simulink model "CaseD_2"  (R2015a)
settings: Solver=ode3  SolverMode=SingleTasking  StartTime=0.0  StopTime=time  FixedStep=dt  RelTol=1e-3
values from neighbouring files (symbols this model uses):
  C = [6; 0]    [main.m]
  dt = 0.01    [main.m]
  initial_eta = [1 0 0]'    [main.m]
  initial_eta_2 = [6 5 0]'    [main.m]
  initial_eta_4 = [7 0 0]'    [main.m]
  K_p = diag([0.2,0.2,0.1])    [main.m]
  mu = 0.1    [main.m]
  P_d = [2  0 ... (first row only)    [main.m]
  R = diag(r)    [main.m]
  r = [5; 3]    [main.m]
  U_max = 1    [main.m]
  U_ref = [(0:dt:time)' [zeros(floor(1*points/6),1) ... (first row only)    [main.m]
(part 1 of 2)
settings Model: CovMetricSettings=dwe  CovHtmlReporting=off  covSaveCumulativeToWorkspaceVar=off  CovSaveSingleToWorkspaceVar=off  CovExternalEMLEnable=on  Creator=helene  LastModifiedBy=Lars
settings DataIOCC: LimitDataPoints=off  SaveFormat=Dataset
settings DebuggingCC: SFUnexpectedBacktrackingDiag=error  SFNoUnconditionalDefaultTransitionDiag=error
settings HardwareCC: ProdBitPerPointer=64  ProdLargestAtomicFloat=Float  ProdIntDivRoundTo=Zero  ProdEndianess=LittleEndian  ProdHWDeviceType=Specified
settings ModelReferenceCC: PropagateSignalLabelsOutOfModel=on
settings GRTTargetCC: TargetLangStandard=C99 (ISO)  GeneratePreprocessorConditionals=Use local settings

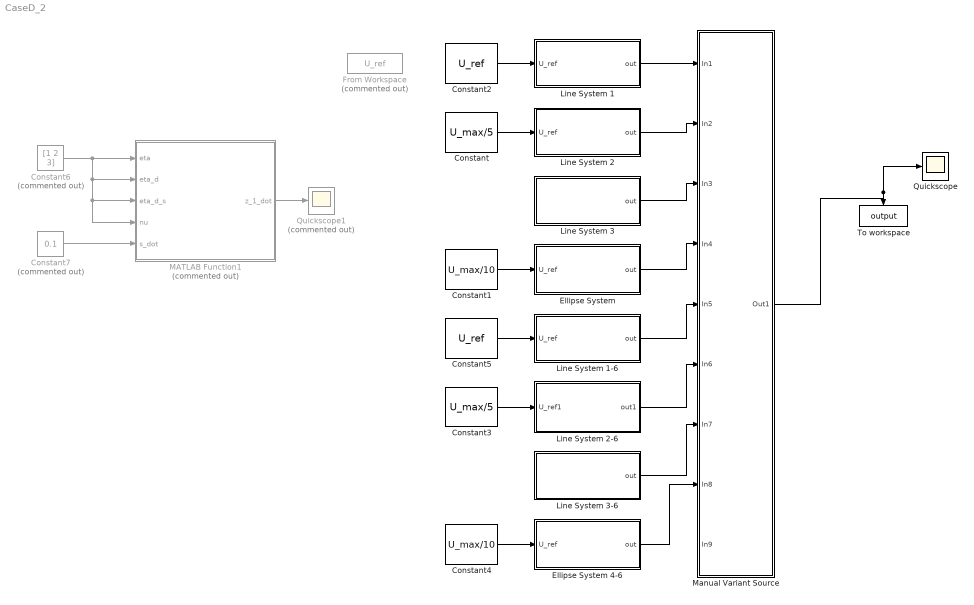
== system CaseD_2 ==
  Constant : Constant  Value=U_max/5
  Constant1 : Constant  Value=U_max/10
  Constant2 : Constant  Value=U_ref
  Constant3 : Constant  Value=U_max/5
  Constant4 : Constant  Value=U_max/10
  Constant5 : Constant  Value=U_ref
  Constant6 : Constant  Commented=on  Value=[1 2 3]
  Constant7 : Constant  Commented=on  Value=0.1
  Ellipse System : Subsystem
  Ellipse System 4-6 : Subsystem
  From Workspace : FromWorkspace  Commented=on  VariableName=U_ref  SampleTime=dt
  Line System 1 : Subsystem
  Line System 1-6 : Subsystem
  Line System 2 : Subsystem
  Line System 2-6 : Subsystem
  Line System 3 : Subsystem
  Line System 3-6 : Subsystem
  MATLAB Function1 : MATLAB Function  Commented=on  TreatAsAtomicUnit=on
      settings: PermitHierarchicalResolution=ParametersOnly
  Manual Variant Source : Subsystem  Description=Replaced Block  mask(Replaced Block){}
      mask help: This block has been replaced with an empty subsystem because it used functionality that is unavailable in Simulink R2015a.
      mask Display: fprintf('Replaced: %s\n','VariantSource')
  Quickscope : Scope
      settings: TimeRange=auto  ShowLegends=on  MaxDataPoints=5000  SaveToWorkspace=off  YMin=-2.04605  YMax=18.41446  SampleTime=-1
  Quickscope1 : Scope  Commented=on
      settings: TimeRange=auto  MaxDataPoints=5000  SaveToWorkspace=off  YMin=0.86712  YMax=2.90365  SampleTime=-1
  To workspace : ToWorkspace  VariableName=output  SampleTime=-1
      settings: StopFcn=plotting
  wires:
  Ellipse System/1(out) -> Manual Variant Source/4(In4)
  Manual Variant Source/1(Out1) -> Quickscope/1, To workspace/1
  Line System 1/1(out) -> Manual Variant Source/1(In1)
  Line System 2/1(out) -> Manual Variant Source/2(In2)
  Constant/1 -> Line System 2/1(U_ref)
  Line System 3/1(out) -> Manual Variant Source/3(In3)
  Constant1/1 -> Ellipse System/1(U_ref)
  Constant2/1 -> Line System 1/1(U_ref)
  Ellipse System 4-6/1(out) -> Manual Variant Source/8(In8)
  Line System 1-6/1(out) -> Manual Variant Source/5(In5)
  Line System 2-6/1(out1) -> Manual Variant Source/6(In6)
  Constant3/1 -> Line System 2-6/1(U_ref1)
  Line System 3-6/1(out) -> Manual Variant Source/7(In7)
  Constant4/1 -> Ellipse System 4-6/1(U_ref)
  Constant5/1 -> Line System 1-6/1(U_ref)
  Constant6/1 -> MATLAB Function1/4(nu), MATLAB Function1/3(eta_d_s), MATLAB Function1/2(eta_d), MATLAB Function1/1(eta)
  Constant7/1 -> MATLAB Function1/5(s_dot)
  MATLAB Function1/1(z_1_dot) -> Quickscope1/1

== system CaseD_2/Ellipse System ==
  U_ref : Inport
  Control law : Subsystem
  "Ellipse Mapper " : Subsystem
  Ellipse Speed Gauge : Subsystem
  Kinematic model : Subsystem
  Mux : Mux  Inputs=3
  Update Law : Subsystem
  out : Outport
  wires:
  U_ref/1 -> Ellipse Speed Gauge/1(U_ref)
  Update Law/1(s) -> Mux/3, Ellipse Speed Gauge/2(s), "Ellipse Mapper "/1(s)
  "Ellipse Mapper "/1(eta_d) -> Update Law/2(eta_d), Mux/2, Control law/4(eta_d)
  Kinematic model/1("eta ") -> Control law/1(eta), Update Law/4(eta), Mux/1
  Control law/1(nu) -> Kinematic model/1(nu)
  "Ellipse Mapper "/2(eta_d_s) -> Control law/3(eta_d_s), Update Law/3(eta_d_s)
  Ellipse Speed Gauge/1(U_s) -> Control law/2(U_s), Update Law/1(U_s)
  Mux/1 -> out/1

== system CaseD_2/Ellipse System 4-6 ==
  U_ref : Inport
  Control law1 : Subsystem
  "Ellipse Mapper " : Subsystem
  Ellipse Speed Gauge : Subsystem
  Kinematic model : Subsystem
  Mux : Mux  Inputs=3
  Update Law : Subsystem
  out : Outport
  wires:
  U_ref/1 -> Ellipse Speed Gauge/1(U_ref)
  Update Law/1(s) -> Ellipse Speed Gauge/2(s), "Ellipse Mapper "/1(s), Mux/3
  "Ellipse Mapper "/1(eta_d) -> Control law1/3(eta_d), Update Law/2(eta_d), Mux/2
  Kinematic model/1("eta ") -> Control law1/7(eta), Update Law/4(eta), Mux/1
  Control law1/1(new_nu) -> Control law1/8(nu), Kinematic model/1(nu)
  "Ellipse Mapper "/2(eta_d_s) -> Update Law/3(eta_d_s), Control law1/2(eta_d_s)
  Ellipse Speed Gauge/1(U_s) -> Control law1/1(U_s), Update Law/1(U_s)
  Mux/1 -> out/1
  Update Law/2(s_dot) -> Control law1/4(s_dot)
  Ellipse Speed Gauge/2(U_s_s) -> Control law1/5(U_s_s)
  "Ellipse Mapper "/3(eta_d_ss) -> Control law1/6(eta_d_ss)

== system CaseD_2/Line System 1 ==
  U_ref : Inport
  Control law : Subsystem
  Kinematic model : Subsystem
  Line Mapper : Subsystem
  Line Speed Gauge : Subsystem
  Mux : Mux  Inputs=3
  Update Law : Subsystem
  out : Outport
  wires:
  U_ref/1 -> Line Speed Gauge/1(U_ref)
  Update Law/1(s) -> Mux/3, Line Mapper/1("s ")
  Control law/1(nu) -> Kinematic model/1(nu)
  Line Mapper/2(eta_d_s) -> Control law/3(eta_d_s), Update Law/3(eta_d_s)
  Line Speed Gauge/1(U_s) -> Control law/2(U_s), Update Law/1(U_s)
  Line Mapper/1(eta_d) -> Control law/4(eta_d), Update Law/2(eta_d), Mux/2
  Kinematic model/1("eta ") -> Control law/1(eta), Update Law/4(eta), Mux/1
  Mux/1 -> out/1

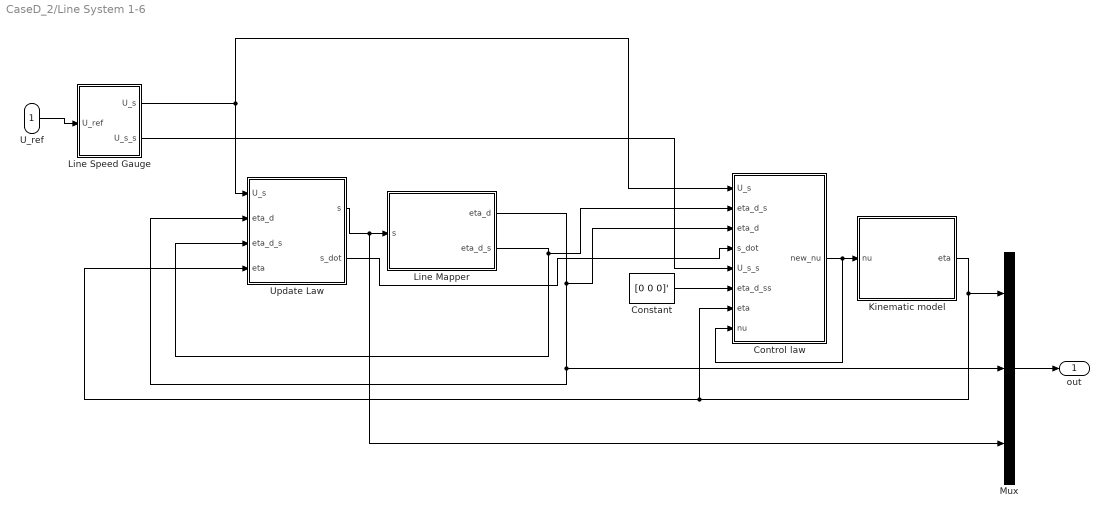
== system CaseD_2/Line System 1-6 ==
  U_ref : Inport
  Constant : Constant  Value=[0 0 0]'
  Control law : Subsystem
  Kinematic model : Subsystem
  Line Mapper : Subsystem
  Line Speed Gauge : Subsystem
  Mux : Mux  Inputs=3
  Update Law : Subsystem
  out : Outport
  wires:
  U_ref/1 -> Line Speed Gauge/1(U_ref)
  Update Law/1(s) -> Mux/3, Line Mapper/1("s ")
  Control law/1(new_nu) -> Control law/8(nu), Kinematic model/1(nu)
  Line Mapper/2(eta_d_s) -> Control law/2(eta_d_s), Update Law/3(eta_d_s)
  Line Speed Gauge/1(U_s) -> Control law/1(U_s), Update Law/1(U_s)
  Line Mapper/1(eta_d) -> Control law/3(eta_d), Update Law/2(eta_d), Mux/2
  Kinematic model/1("eta ") -> Control law/7(eta), Update Law/4(eta), Mux/1
  Mux/1 -> out/1
  Update Law/2(s_dot) -> Control law/4(s_dot)
  Line Speed Gauge/2(U_s_s) -> Control law/5(U_s_s)
  Constant/1 -> Control law/6(eta_d_ss)

== system CaseD_2/Line System 2 ==
  U_ref : Inport
  Control law : Subsystem
  Kinematic model : Subsystem
  Line Mapper : Subsystem
  Line Speed Gauge : Subsystem
  Mux : Mux  Inputs=3
  Update Law : Subsystem
  out : Outport
  wires:
  U_ref/1 -> Line Speed Gauge/1(U_ref)
  Update Law/1(s) -> Mux/3, Line Mapper/1("s ")
  Control law/1(nu) -> Kinematic model/1(nu)
  Line Mapper/2(eta_d_s) -> Update Law/3(eta_d_s), Control law/3(eta_d_s)
  Line Speed Gauge/1(U_s) -> Control law/2(U_s), Update Law/1(U_s)
  Line Mapper/1(eta_d) -> Update Law/2(eta_d), Mux/2, Control law/4(eta_d)
  Kinematic model/1("eta ") -> Control law/1(eta), Update Law/4(eta), Mux/1
  Mux/1 -> out/1

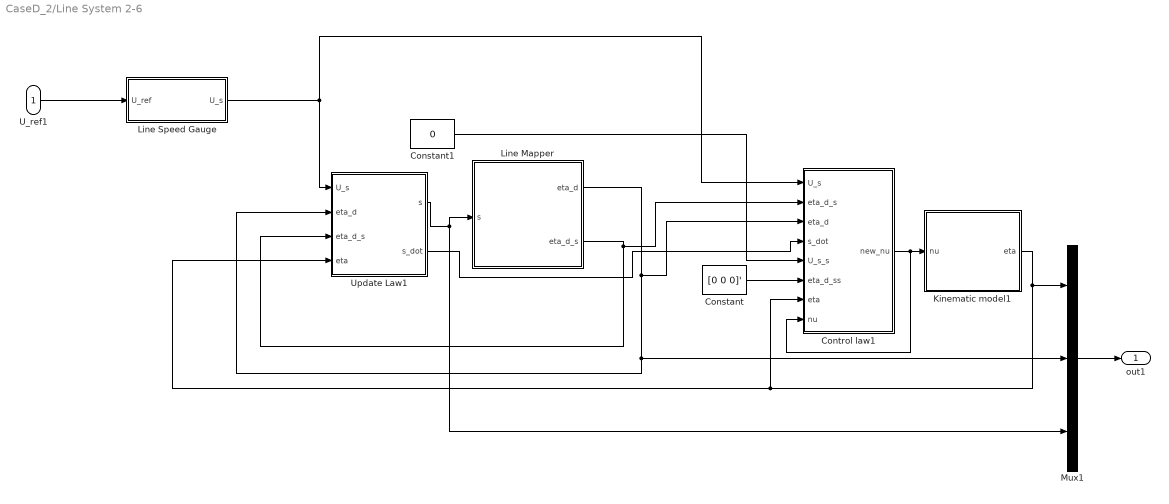
== system CaseD_2/Line System 2-6 ==
  U_ref1 : Inport
  Constant : Constant  Value=[0 0 0]'
  Constant1 : Constant  Value=0
  Control law1 : Subsystem
  Kinematic model1 : Subsystem
  Line Mapper : Subsystem
  Line Speed Gauge : Subsystem
  Mux1 : Mux  Inputs=3
  Update Law1 : Subsystem
  out1 : Outport
  wires:
  U_ref1/1 -> Line Speed Gauge/1(U_ref)
  Update Law1/1(s) -> Line Mapper/1("s "), Mux1/3
  Control law1/1(new_nu) -> Control law1/8(nu), Kinematic model1/1(nu)
  Line Mapper/2(eta_d_s) -> Control law1/2(eta_d_s), Update Law1/3(eta_d_s)
  Line Speed Gauge/1(U_s) -> Control law1/1(U_s), Update Law1/1(U_s)
  Line Mapper/1(eta_d) -> Control law1/3(eta_d), Update Law1/2(eta_d), Mux1/2
  Kinematic model1/1("eta ") -> Control law1/7(eta), Update Law1/4(eta), Mux1/1
  Mux1/1 -> out1/1
  Update Law1/2(s_dot) -> Control law1/4(s_dot)
  Constant1/1 -> Control law1/5(U_s_s)
  Constant/1 -> Control law1/6(eta_d_ss)

== system CaseD_2/Line System 3 ==
  Constant1 : Constant  Value=U_max/5
  Control law : Subsystem
  Kinematic model : Subsystem
  Line Mapper : Subsystem
  Line Speed Gauge : Subsystem
  MATLAB Function : MATLAB Function  TreatAsAtomicUnit=on
      settings: PermitHierarchicalResolution=ParametersOnly
  Mux : Mux  Inputs=3
  Update Law : Subsystem
  out : Outport
  wires:
  Update Law/1(s) -> Line Mapper/1(s), Mux/3, MATLAB Function/2(s)
  Control law/1(nu) -> Kinematic model/1(nu)
  Line Mapper/2(eta_d_s) -> Control law/3(eta_d_s), Update Law/3(eta_d_s)
  Line Speed Gauge/1(U_s) -> Control law/2(U_s), Update Law/1(U_s)
  Line Mapper/1(eta_d) -> Control law/4(eta_d), Update Law/2(eta_d), Mux/2
  Kinematic model/1("eta ") -> Control law/1(eta), Update Law/4(eta), Mux/1
  Mux/1 -> out/1
  MATLAB Function/1(U_ref) -> Line Speed Gauge/1(U_ref)
  Constant1/1 -> MATLAB Function/1(scaled_U_max)

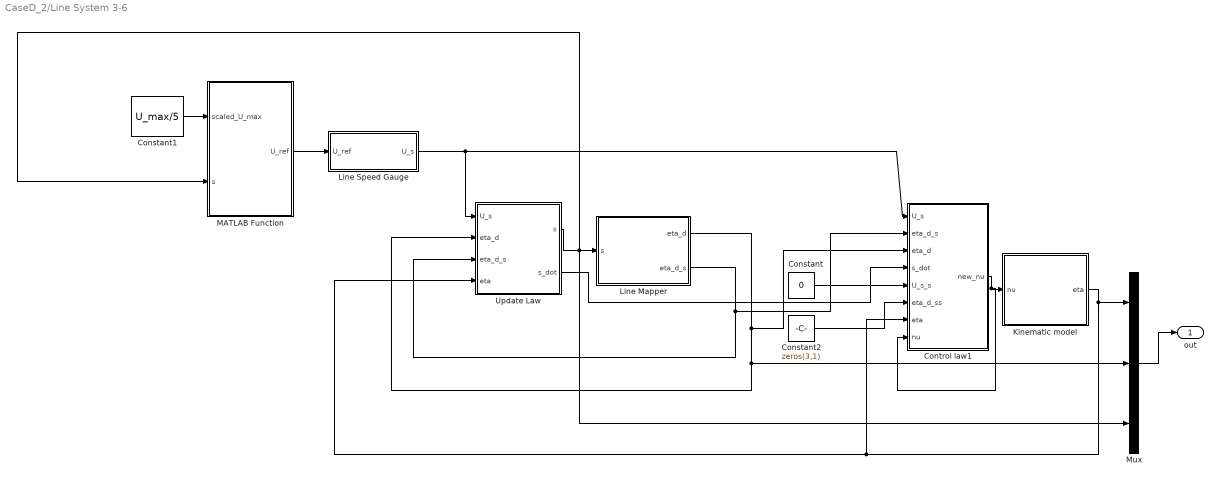
== system CaseD_2/Line System 3-6 ==
  Constant : Constant  Value=0
  Constant1 : Constant  Value=U_max/5
  Constant2 : Constant  Value=zeros(3,1)
  Control law1 : Subsystem
  Kinematic model : Subsystem
  Line Mapper : Subsystem
  Line Speed Gauge : Subsystem
  MATLAB Function : MATLAB Function  TreatAsAtomicUnit=on
      settings: PermitHierarchicalResolution=ParametersOnly
  Mux : Mux  Inputs=3
  Update Law : Subsystem
  out : Outport
  wires:
  Update Law/1(s) -> Line Mapper/1(s), Mux/3, MATLAB Function/2(s)
  Control law1/1(new_nu) -> Control law1/8(nu), Kinematic model/1(nu)
  Line Mapper/2(eta_d_s) -> Control law1/2(eta_d_s), Update Law/3(eta_d_s)
  Line Speed Gauge/1(U_s) -> Control law1/1(U_s), Update Law/1(U_s)
  Line Mapper/1(eta_d) -> Control law1/3(eta_d), Update Law/2(eta_d), Mux/2
  Kinematic model/1("eta ") -> Control law1/7(eta), Update Law/4(eta), Mux/1
  Mux/1 -> out/1
  MATLAB Function/1(U_ref) -> Line Speed Gauge/1(U_ref)
  Constant1/1 -> MATLAB Function/1(scaled_U_max)
  Update Law/2(s_dot) -> Control law1/4(s_dot)
  Constant/1 -> Control law1/5(U_s_s)
  Constant2/1 -> Control law1/6(eta_d_ss)

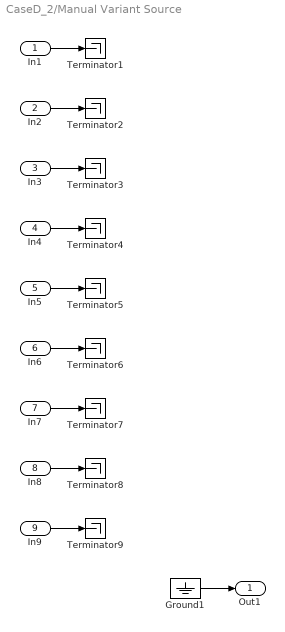
== system CaseD_2/Manual Variant Source ==
  In1 : Inport
  In2 : Inport  Port=2
  In3 : Inport  Port=3
  In4 : Inport  Port=4
  In5 : Inport  Port=5
  In6 : Inport  Port=6
  In7 : Inport  Port=7
  In8 : Inport  Port=8
  In9 : Inport  Port=9
  Ground1 : Ground
  Terminator{1..9} (9 alike) : Terminator
  Out1 : Outport
  wires:
  Ground1/1 -> Out1/1
  In9/1 -> Terminator9/1
  In8/1 -> Terminator8/1
  In7/1 -> Terminator7/1
  In6/1 -> Terminator6/1
  In5/1 -> Terminator5/1
  In4/1 -> Terminator4/1
  In3/1 -> Terminator3/1
  In2/1 -> Terminator2/1
  In1/1 -> Terminator1/1

== system CaseD_2/Ellipse System/Control law ==
  eta : Inport
  U_s : Inport  Port=2
  eta_d_s : Inport  Port=3
  eta_d : Inport  Port=4
  Control Law : MATLAB Function  TreatAsAtomicUnit=on
      settings: PermitHierarchicalResolution=ParametersOnly
  K_p : Constant  Value=K_p
  Scope : Scope
      settings: TimeRange=auto  MaxDataPoints=5000  SaveToWorkspace=off  SaveName=ScopeData3  YMin=-10576.35102  YMax=10326.26692  SampleTime=-1
  nu : Outport
  wires:
  K_p/1 -> Control Law/1(K_p)
  Control Law/1(nu) -> nu/1
  eta_d_s/1 -> Control Law/4(eta_d_s)
  U_s/1 -> Control Law/5(U_s)
  eta_d/1 -> Control Law/3(eta_d)
  eta/1 -> Control Law/2(eta)
  Control Law/2(z_1) -> Scope/1

== system CaseD_2/Ellipse System/Ellipse Mapper  ==
  s : Inport
  Constant : Constant  Value=R
  Constant1 : Constant  Value=C
  Ellipse Mapper : MATLAB Function  TreatAsAtomicUnit=on
      settings: PermitHierarchicalResolution=ParametersOnly
  eta_d : Outport  PortDimensions=3
  eta_d_s : Outport  Port=2  PortDimensions=3
  wires:
  Ellipse Mapper/1(eta_d) -> eta_d/1
  Ellipse Mapper/2(eta_d_s) -> eta_d_s/1
  Constant1/1 -> Ellipse Mapper/2(C)
  Constant/1 -> Ellipse Mapper/3(R)
  s/1 -> Ellipse Mapper/1(s)

== system CaseD_2/Ellipse System/Ellipse Speed Gauge ==
  U_ref : Inport
  s : Inport  Port=2
  Constant : Constant  Value=r
  Ellipse : MATLAB Function  TreatAsAtomicUnit=on
      settings: PermitHierarchicalResolution=ParametersOnly
  U_s : Outport
  wires:
  U_ref/1 -> Ellipse/1(U_ref)
  Ellipse/1(U_s) -> U_s/1
  Constant/1 -> Ellipse/3(r)
  s/1 -> Ellipse/2(s)

== system CaseD_2/Ellipse System/Kinematic model ==
  nu : Inport
  Integrator : Integrator  InitialCondition=initial_eta_4
  MATLAB Function : MATLAB Function  TreatAsAtomicUnit=on
      settings: PermitHierarchicalResolution=ParametersOnly
  Product : Product  Multiplication=Matrix(*)
  Rotation matrix : MATLAB Function  TreatAsAtomicUnit=on
      settings: PermitHierarchicalResolution=ParametersOnly
  Selector : Selector  InputPortWidth=3  IndexOptions=Starting index (dialog)  Indices=3  OutputSizes=1
  "eta " : Outport
  wires:
  Product/1 -> Integrator/1  "eta_dot"
  Integrator/1 -> MATLAB Function/1("eta "), Selector/1  "eta"
  nu/1 -> Product/2
  Rotation matrix/1(R) -> Product/1
  Selector/1 -> Rotation matrix/1(psi)
  MATLAB Function/1(eta) -> "eta "/1

== system CaseD_2/Ellipse System/Update Law ==
  U_s : Inport
  eta_d : Inport  Port=2
  eta_d_s : Inport  Port=3
  eta : Inport  Port=4
  Constant : Constant  Value=mu
  Integrator : Integrator
  Saturation : Saturate  UpperLimit=inf  LowerLimit=0
  Update Law : MATLAB Function  TreatAsAtomicUnit=on
      settings: PermitHierarchicalResolution=ParametersOnly
  s : Outport
  wires:
  U_s/1 -> Update Law/1(U_s)
  Constant/1 -> Update Law/2(mu)
  eta_d_s/1 -> Update Law/3(eta_d_s)
  eta_d/1 -> Update Law/4(eta_d)
  Integrator/1 -> s/1
  eta/1 -> Update Law/5(eta)
  Saturation/1 -> Integrator/1
  Update Law/1(s_dot) -> Saturation/1

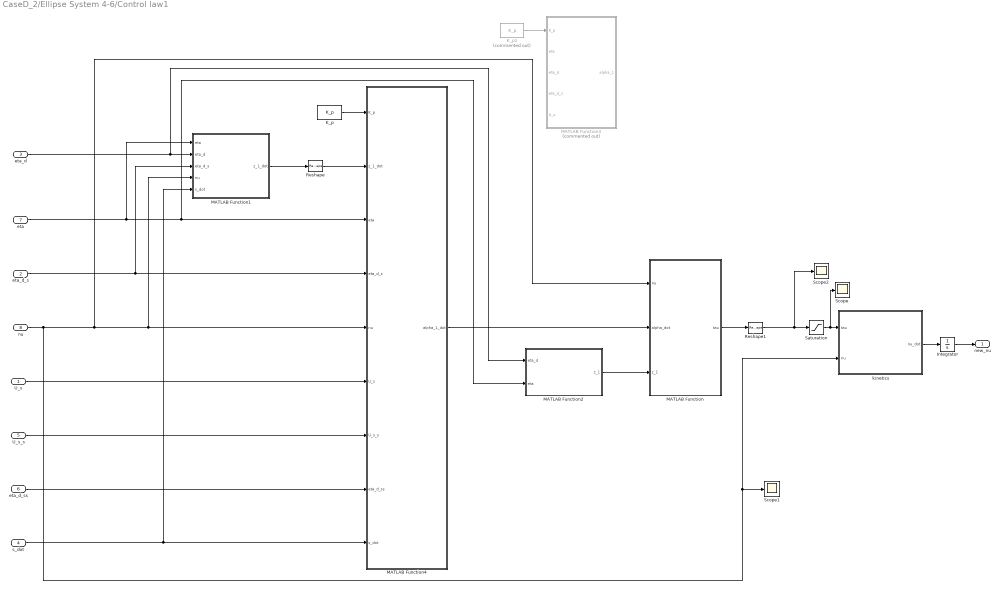
== system CaseD_2/Ellipse System 4-6/Control law1 ==
  U_s : Inport
  eta_d_s : Inport  Port=2
  eta_d : Inport  Port=3
  s_dot : Inport  Port=4
  U_s_s : Inport  Port=5
  eta_d_ss : Inport  Port=6
  eta : Inport  Port=7
  nu : Inport  Port=8
  Integrator : Integrator  InitialCondition=[0 0 0]'
  K_p : Constant  Value=K_p
  K_p1 : Constant  Commented=on  Value=K_p
  MATLAB Function : MATLAB Function  TreatAsAtomicUnit=on
      settings: PermitHierarchicalResolution=ParametersOnly
  MATLAB Function1 : MATLAB Function  TreatAsAtomicUnit=on
      settings: PermitHierarchicalResolution=ParametersOnly
  MATLAB Function2 : MATLAB Function  TreatAsAtomicUnit=on
      settings: PermitHierarchicalResolution=ParametersOnly
  MATLAB Function3 : MATLAB Function  Commented=on  TreatAsAtomicUnit=on
      settings: PermitHierarchicalResolution=ParametersOnly
  MATLAB Function4 : MATLAB Function  TreatAsAtomicUnit=on
      settings: PermitHierarchicalResolution=ParametersOnly
  Reshape : Reshape  OutputDimensionality=Customize  OutputDimensions=[3,1]
  Reshape1 : Reshape  OutputDimensionality=Customize  OutputDimensions=[3,1]
  Saturation : Saturate  UpperLimit=[1.03 2.5 0.98]'  LowerLimit=-[1.03 2.5 0.98]'
  Scope : Scope
      settings: TimeRange=auto  ShowLegends=on  MaxDataPoints=5000  SaveToWorkspace=off  YMin=-3.125  YMax=3.125  SampleTime=-1
  Scope1 : Scope
      settings: TimeRange=auto  MaxDataPoints=5000  SaveToWorkspace=off  SaveName=ScopeData2  YMin=-4361622909727543.00000  YMax=330140861095278.5  SampleTime=-1
  Scope2 : Scope
      settings: TimeRange=auto  MaxDataPoints=5000  SaveToWorkspace=off  SaveName=ScopeData3  YMin=-65.86026  YMax=75.79879  SampleTime=-1
  kinetics : MATLAB Function  TreatAsAtomicUnit=on
      settings: PermitHierarchicalResolution=ParametersOnly
  new_nu : Outport
  wires:
  eta_d_s/1 -> MATLAB Function1/3(eta_d_s), MATLAB Function4/4(eta_d_s)
  U_s/1 -> MATLAB Function4/6(U_s)
  eta_d/1 -> MATLAB Function2/1(eta_d), MATLAB Function1/2(eta_d)
  eta/1 -> MATLAB Function1/1(eta), MATLAB Function2/2(eta), MATLAB Function4/3(eta)
  MATLAB Function/1(tau) -> Reshape1/1
  K_p1/1 -> MATLAB Function3/1(K_p)
  MATLAB Function4/1(alpha_1_dot) -> MATLAB Function/2(alpha_dot)
  MATLAB Function1/1(z_1_dot) -> Reshape/1
  K_p/1 -> MATLAB Function4/1(K_p)
  U_s_s/1 -> MATLAB Function4/7(U_s_s)
  eta_d_ss/1 -> MATLAB Function4/8(eta_d_ss)
  s_dot/1 -> MATLAB Function1/5(s_dot), MATLAB Function4/9(s_dot)
  MATLAB Function2/1(z_1) -> MATLAB Function/3(z_1)
  Integrator/1 -> new_nu/1
  kinetics/1(nu_dot) -> Integrator/1
  nu/1 -> Scope1/1, kinetics/2(nu), MATLAB Function/1(nu), MATLAB Function1/4(nu), MATLAB Function4/5(nu)
  Saturation/1 -> Scope/1, kinetics/1(tau)
  Reshape/1 -> MATLAB Function4/2(z_1_dot)
  Reshape1/1 -> Scope2/1, Saturation/1

== system CaseD_2/Ellipse System 4-6/Ellipse Mapper  ==
  s : Inport
  Constant : Constant  Value=R
  Constant1 : Constant  Value=C
  Ellipse Mapper : MATLAB Function  TreatAsAtomicUnit=on
      settings: PermitHierarchicalResolution=ParametersOnly
  eta_d : Outport  PortDimensions=3
  eta_d_s : Outport  Port=2  PortDimensions=3
  eta_d_ss : Outport  Port=3  PortDimensions=3
  wires:
  Ellipse Mapper/1(eta_d) -> eta_d/1
  Ellipse Mapper/2(eta_d_s) -> eta_d_s/1
  Constant1/1 -> Ellipse Mapper/2(C)
  Constant/1 -> Ellipse Mapper/3(R)
  s/1 -> Ellipse Mapper/1(s)
  Ellipse Mapper/3(eta_d_ss) -> eta_d_ss/1

== system CaseD_2/Ellipse System 4-6/Ellipse Speed Gauge ==
  U_ref : Inport
  s : Inport  Port=2
  Constant : Constant  Value=r
  Ellipse : MATLAB Function  TreatAsAtomicUnit=on
      settings: PermitHierarchicalResolution=ParametersOnly
  U_s : Outport
  U_s_s : Outport  Port=2
  wires:
  U_ref/1 -> Ellipse/1(U_ref)
  Ellipse/1(U_s) -> U_s/1
  Constant/1 -> Ellipse/3(r)
  s/1 -> Ellipse/2(s)
  Ellipse/2(U_s_s) -> U_s_s/1

== system CaseD_2/Ellipse System 4-6/Kinematic model ==
  nu : Inport
  Integrator : Integrator  InitialCondition=initial_eta_4
  MATLAB Function : MATLAB Function  TreatAsAtomicUnit=on
      settings: PermitHierarchicalResolution=ParametersOnly
  Product : Product  Multiplication=Matrix(*)
  Rotation matrix : MATLAB Function  TreatAsAtomicUnit=on
      settings: PermitHierarchicalResolution=ParametersOnly
  Selector : Selector  InputPortWidth=3  IndexOptions=Starting index (dialog)  Indices=3  OutputSizes=1
  "eta " : Outport
  wires:
  Product/1 -> Integrator/1  "eta_dot"
  Integrator/1 -> MATLAB Function/1("eta "), Selector/1  "eta"
  nu/1 -> Product/2
  Rotation matrix/1(R) -> Product/1
  Selector/1 -> Rotation matrix/1(psi)
  MATLAB Function/1(eta) -> "eta "/1

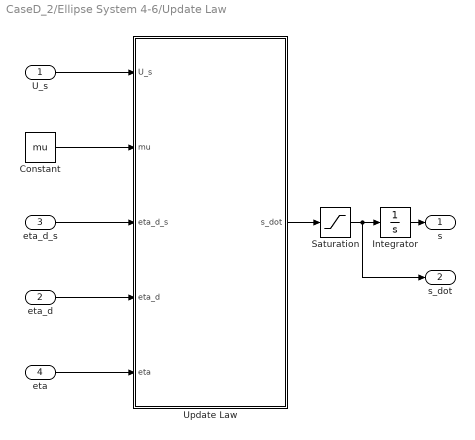
== system CaseD_2/Ellipse System 4-6/Update Law ==
  U_s : Inport
  eta_d : Inport  Port=2
  eta_d_s : Inport  Port=3
  eta : Inport  Port=4
  Constant : Constant  Value=mu
  Integrator : Integrator
  Saturation : Saturate  UpperLimit=inf  LowerLimit=0
  Update Law : MATLAB Function  TreatAsAtomicUnit=on
      settings: PermitHierarchicalResolution=ParametersOnly
  s : Outport
  s_dot : Outport  Port=2
  wires:
  U_s/1 -> Update Law/1(U_s)
  Constant/1 -> Update Law/2(mu)
  eta_d_s/1 -> Update Law/3(eta_d_s)
  eta_d/1 -> Update Law/4(eta_d)
  Integrator/1 -> s/1
  eta/1 -> Update Law/5(eta)
  Saturation/1 -> s_dot/1, Integrator/1
  Update Law/1(s_dot) -> Saturation/1

== system CaseD_2/Line System 1/Control law ==
  eta : Inport
  U_s : Inport  Port=2
  eta_d_s : Inport  Port=3
  eta_d : Inport  Port=4
  Control Law : MATLAB Function  TreatAsAtomicUnit=on
      settings: PermitHierarchicalResolution=ParametersOnly
  K_p : Constant  Value=K_p
  Scope : Scope
      settings: TimeRange=auto  MaxDataPoints=5000  SaveToWorkspace=off  SaveName=ScopeData3  YMin=-10576.35102  YMax=10326.26692  SampleTime=-1
  nu : Outport
  wires:
  K_p/1 -> Control Law/1(K_p)
  Control Law/1(nu) -> nu/1
  eta_d_s/1 -> Control Law/4(eta_d_s)
  U_s/1 -> Control Law/5(U_s)
  eta_d/1 -> Control Law/3(eta_d)
  eta/1 -> Control Law/2(eta)
  Control Law/2(z_1) -> Scope/1

== system CaseD_2/Line System 1/Kinematic model ==
  nu : Inport
  Integrator : Integrator  InitialCondition=initial_eta
  Product : Product  Multiplication=Matrix(*)
  Rotation matrix : MATLAB Function  TreatAsAtomicUnit=on
      settings: PermitHierarchicalResolution=ParametersOnly
  Selector : Selector  InputPortWidth=3  IndexOptions=Starting index (dialog)  Indices=3  OutputSizes=1
  "eta " : Outport
  wires:
  Product/1 -> Integrator/1  "eta_dot"
  Integrator/1 -> Selector/1, "eta "/1  "eta"
  nu/1 -> Product/2
  Rotation matrix/1(R) -> Product/1
  Selector/1 -> Rotation matrix/1(psi)

== system CaseD_2/Line System 1/Line Mapper ==
  "s " : Inport
  MATLAB Function : MATLAB Function  TreatAsAtomicUnit=on
      settings: PermitHierarchicalResolution=ParametersOnly
  P_d : Constant  Value=P_d
  eta_d : Outport  PortDimensions=3
  eta_d_s : Outport  Port=2  PortDimensions=3
  wires:
  MATLAB Function/1(eta_d) -> eta_d/1
  MATLAB Function/2(eta_d_s) -> eta_d_s/1
  "s "/1 -> MATLAB Function/1(s)
  P_d/1 -> MATLAB Function/2(P_d)

== system CaseD_2/Line System 1/Line Speed Gauge ==
  U_ref : Inport
  Constant : Constant  Value=P_d
  Line : MATLAB Function  TreatAsAtomicUnit=on
      settings: PermitHierarchicalResolution=ParametersOnly
  U_s : Outport
  wires:
  U_ref/1 -> Line/1(U_ref)
  Line/1(U_s) -> U_s/1
  Constant/1 -> Line/2(P_d)

== system CaseD_2/Line System 1/Update Law ==
  U_s : Inport
  eta_d : Inport  Port=2
  eta_d_s : Inport  Port=3
  eta : Inport  Port=4
  Constant : Constant  Value=mu
  Integrator : Integrator  LimitOutput=on  UpperSaturationLimit=1  LowerSaturationLimit=0
  Update Law : MATLAB Function  TreatAsAtomicUnit=on
      settings: PermitHierarchicalResolution=ParametersOnly
  s : Outport
  wires:
  U_s/1 -> Update Law/1(U_s)
  Constant/1 -> Update Law/2(mu)
  eta_d_s/1 -> Update Law/3(eta_d_s)
  eta_d/1 -> Update Law/4(eta_d)
  Update Law/1(s_dot) -> Integrator/1
  Integrator/1 -> s/1
  eta/1 -> Update Law/5(eta)

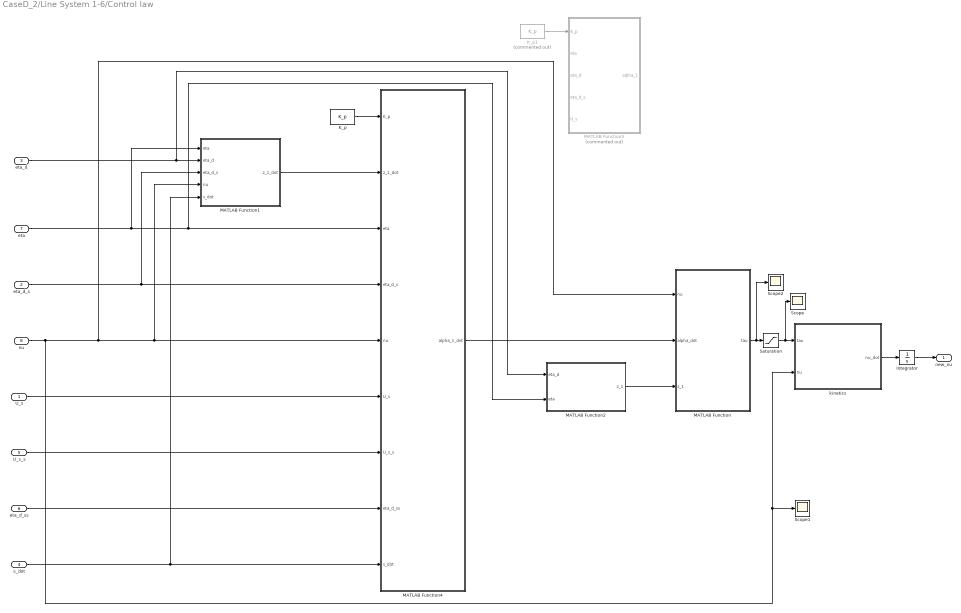
== system CaseD_2/Line System 1-6/Control law ==
  U_s : Inport
  eta_d_s : Inport  Port=2
  eta_d : Inport  Port=3
  s_dot : Inport  Port=4
  U_s_s : Inport  Port=5
  eta_d_ss : Inport  Port=6
  eta : Inport  Port=7
  nu : Inport  Port=8
  Integrator : Integrator  InitialCondition=[0 0 0]'
  K_p : Constant  Value=K_p
  K_p1 : Constant  Commented=on  Value=K_p
  MATLAB Function : MATLAB Function  TreatAsAtomicUnit=on
      settings: PermitHierarchicalResolution=ParametersOnly
  MATLAB Function1 : MATLAB Function  TreatAsAtomicUnit=on
      settings: PermitHierarchicalResolution=ParametersOnly
  MATLAB Function2 : MATLAB Function  TreatAsAtomicUnit=on
      settings: PermitHierarchicalResolution=ParametersOnly
  MATLAB Function3 : MATLAB Function  Commented=on  TreatAsAtomicUnit=on
      settings: PermitHierarchicalResolution=ParametersOnly
  MATLAB Function4 : MATLAB Function  TreatAsAtomicUnit=on
      settings: PermitHierarchicalResolution=ParametersOnly
  Saturation : Saturate  UpperLimit=[1.03 2.5 0.98]'  LowerLimit=-[1.03 2.5 0.98]'
  Scope : Scope
      settings: TimeRange=auto  ShowLegends=on  MaxDataPoints=5000  SaveToWorkspace=off  YMin=-3.125  YMax=3.125  SampleTime=-1
  Scope1 : Scope
      settings: TimeRange=auto  MaxDataPoints=5000  SaveToWorkspace=off  SaveName=ScopeData2  YMin=-4361622909727543.00000  YMax=330140861095278.5  SampleTime=-1
  Scope2 : Scope
      settings: TimeRange=auto  MaxDataPoints=5000  SaveToWorkspace=off  SaveName=ScopeData3  YMin=-65.86026  YMax=75.79879  SampleTime=-1
  kinetics : MATLAB Function  TreatAsAtomicUnit=on
      settings: PermitHierarchicalResolution=ParametersOnly
  new_nu : Outport
  wires:
  eta_d_s/1 -> MATLAB Function1/3(eta_d_s), MATLAB Function4/4(eta_d_s)
  U_s/1 -> MATLAB Function4/6(U_s)
  eta_d/1 -> MATLAB Function2/1(eta_d), MATLAB Function1/2(eta_d)
  eta/1 -> MATLAB Function1/1(eta), MATLAB Function2/2(eta), MATLAB Function4/3(eta)
  MATLAB Function/1(tau) -> Scope2/1, Saturation/1
  K_p1/1 -> MATLAB Function3/1(K_p)
  MATLAB Function4/1(alpha_1_dot) -> MATLAB Function/2(alpha_dot)
  MATLAB Function1/1(z_1_dot) -> MATLAB Function4/2(z_1_dot)
  K_p/1 -> MATLAB Function4/1(K_p)
  U_s_s/1 -> MATLAB Function4/7(U_s_s)
  eta_d_ss/1 -> MATLAB Function4/8(eta_d_ss)
  s_dot/1 -> MATLAB Function1/5(s_dot), MATLAB Function4/9(s_dot)
  MATLAB Function2/1(z_1) -> MATLAB Function/3(z_1)
  Integrator/1 -> new_nu/1
  kinetics/1(nu_dot) -> Integrator/1
  nu/1 -> Scope1/1, kinetics/2(nu), MATLAB Function/1(nu), MATLAB Function1/4(nu), MATLAB Function4/5(nu)
  Saturation/1 -> Scope/1, kinetics/1(tau)

== system CaseD_2/Line System 1-6/Kinematic model ==
  nu : Inport
  Integrator : Integrator  InitialCondition=initial_eta
  Product : Product  Multiplication=Matrix(*)
  Rotation matrix : MATLAB Function  TreatAsAtomicUnit=on
      settings: PermitHierarchicalResolution=ParametersOnly
  Selector : Selector  InputPortWidth=3  IndexOptions=Starting index (dialog)  Indices=3  OutputSizes=1
  "eta " : Outport
  wires:
  Product/1 -> Integrator/1  "eta_dot"
  Integrator/1 -> Selector/1, "eta "/1  "eta"
  nu/1 -> Product/2
  Rotation matrix/1(R) -> Product/1
  Selector/1 -> Rotation matrix/1(psi)

== system CaseD_2/Line System 1-6/Line Mapper ==
  "s " : Inport
  MATLAB Function : MATLAB Function  TreatAsAtomicUnit=on
      settings: PermitHierarchicalResolution=ParametersOnly
  P_d : Constant  Value=P_d
  eta_d : Outport  PortDimensions=3
  eta_d_s : Outport  Port=2  PortDimensions=3
  wires:
  MATLAB Function/1(eta_d) -> eta_d/1
  MATLAB Function/2(eta_d_s) -> eta_d_s/1
  "s "/1 -> MATLAB Function/1(s)
  P_d/1 -> MATLAB Function/2(P_d)

== system CaseD_2/Line System 1-6/Line Speed Gauge ==
  U_ref : Inport
  Constant : Constant  Value=P_d
  Line : MATLAB Function  TreatAsAtomicUnit=on
      settings: PermitHierarchicalResolution=ParametersOnly
  U_s : Outport
  U_s_s : Outport  Port=2
  wires:
  U_ref/1 -> Line/1(U_ref)
  Line/1(U_s) -> U_s/1
  Constant/1 -> Line/2(P_d)
  Line/2(U_s_s) -> U_s_s/1

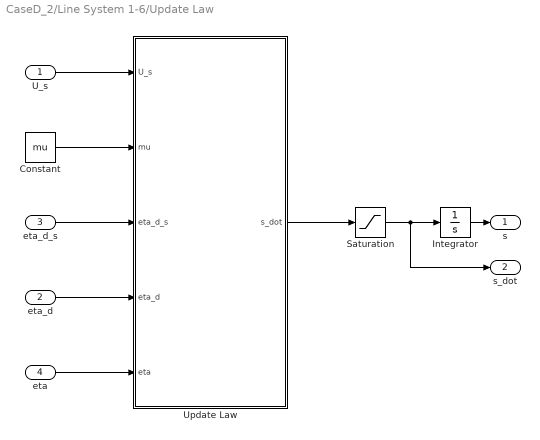
== system CaseD_2/Line System 1-6/Update Law ==
  U_s : Inport
  eta_d : Inport  Port=2
  eta_d_s : Inport  Port=3
  eta : Inport  Port=4
  Constant : Constant  Value=mu
  Integrator : Integrator  LimitOutput=on  UpperSaturationLimit=1  LowerSaturationLimit=0
  Saturation : Saturate  UpperLimit=inf  LowerLimit=0
  Update Law : MATLAB Function  TreatAsAtomicUnit=on
      settings: PermitHierarchicalResolution=ParametersOnly
  s : Outport
  s_dot : Outport  Port=2
  wires:
  U_s/1 -> Update Law/1(U_s)
  Constant/1 -> Update Law/2(mu)
  eta_d_s/1 -> Update Law/3(eta_d_s)
  eta_d/1 -> Update Law/4(eta_d)
  Integrator/1 -> s/1
  eta/1 -> Update Law/5(eta)
  Update Law/1(s_dot) -> Saturation/1
  Saturation/1 -> s_dot/1, Integrator/1

== system CaseD_2/Line System 2/Control law ==
  eta : Inport
  U_s : Inport  Port=2
  eta_d_s : Inport  Port=3
  eta_d : Inport  Port=4
  Control Law : MATLAB Function  TreatAsAtomicUnit=on
      settings: PermitHierarchicalResolution=ParametersOnly
  K_p : Constant  Value=K_p
  Scope : Scope
      settings: TimeRange=auto  MaxDataPoints=5000  SaveToWorkspace=off  SaveName=ScopeData3  YMin=-10576.35102  YMax=10326.26692  SampleTime=-1
  nu : Outport
  wires:
  K_p/1 -> Control Law/1(K_p)
  Control Law/1(nu) -> nu/1
  eta_d_s/1 -> Control Law/4(eta_d_s)
  U_s/1 -> Control Law/5(U_s)
  eta_d/1 -> Control Law/3(eta_d)
  eta/1 -> Control Law/2(eta)
  Control Law/2(z_1) -> Scope/1

== system CaseD_2/Line System 2/Kinematic model ==
  nu : Inport
  Integrator : Integrator  InitialCondition=initial_eta_2
  Product : Product  Multiplication=Matrix(*)
  Rotation matrix : MATLAB Function  TreatAsAtomicUnit=on
      settings: PermitHierarchicalResolution=ParametersOnly
  Selector : Selector  InputPortWidth=3  IndexOptions=Starting index (dialog)  Indices=3  OutputSizes=1
  "eta " : Outport
  wires:
  Product/1 -> Integrator/1  "eta_dot"
  Integrator/1 -> Selector/1, "eta "/1  "eta"
  nu/1 -> Product/2
  Rotation matrix/1(R) -> Product/1
  Selector/1 -> Rotation matrix/1(psi)

== system CaseD_2/Line System 2/Line Mapper ==
  "s " : Inport
  MATLAB Function : MATLAB Function  TreatAsAtomicUnit=on
      settings: PermitHierarchicalResolution=ParametersOnly
  Memory : Memory
  P_d : Constant  Value=P_d
  eta_d : Outport  PortDimensions=3
  eta_d_s : Outport  Port=2  PortDimensions=3
  wires:
  MATLAB Function/1(eta_d) -> eta_d/1
  MATLAB Function/2(eta_d_s) -> eta_d_s/1
  "s "/1 -> MATLAB Function/1(s)
  P_d/1 -> MATLAB Function/2(P_d)
  Memory/1 -> MATLAB Function/3(s_proc_old)
  MATLAB Function/3(s_proc) -> Memory/1

== system CaseD_2/Line System 2/Line Speed Gauge ==
  U_ref : Inport
  Constant : Constant  Value=P_d
  Line : MATLAB Function  TreatAsAtomicUnit=on
      settings: PermitHierarchicalResolution=ParametersOnly
  U_s : Outport
  wires:
  U_ref/1 -> Line/1(U_ref)
  Line/1(U_s) -> U_s/1
  Constant/1 -> Line/2(P_d)

== system CaseD_2/Line System 2/Update Law ==
  U_s : Inport
  eta_d : Inport  Port=2
  eta_d_s : Inport  Port=3
  eta : Inport  Port=4
  Constant : Constant  Value=mu
  Integrator : Integrator  UpperSaturationLimit=1  LowerSaturationLimit=0
  Update Law : MATLAB Function  TreatAsAtomicUnit=on
      settings: PermitHierarchicalResolution=ParametersOnly
  s : Outport
  wires:
  U_s/1 -> Update Law/1(U_s)
  Constant/1 -> Update Law/2(mu)
  eta_d_s/1 -> Update Law/3(eta_d_s)
  eta_d/1 -> Update Law/4(eta_d)
  Integrator/1 -> s/1
  eta/1 -> Update Law/5(eta)
  Update Law/1(s_dot) -> Integrator/1

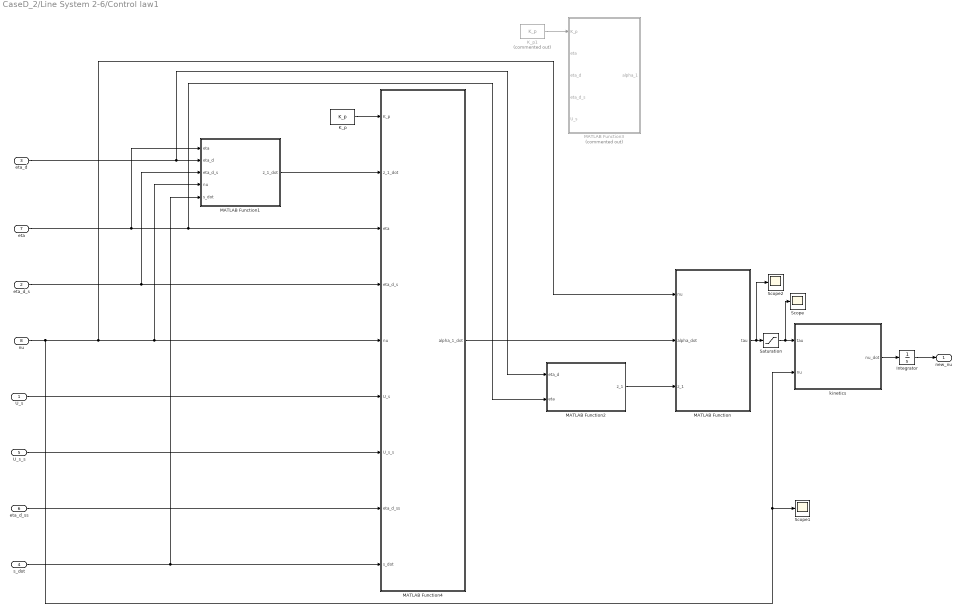
== system CaseD_2/Line System 2-6/Control law1 ==
  U_s : Inport
  eta_d_s : Inport  Port=2
  eta_d : Inport  Port=3
  s_dot : Inport  Port=4
  U_s_s : Inport  Port=5
  eta_d_ss : Inport  Port=6
  eta : Inport  Port=7
  nu : Inport  Port=8
  Integrator : Integrator  InitialCondition=[0 0 0]'
  K_p : Constant  Value=K_p
  K_p1 : Constant  Commented=on  Value=K_p
  MATLAB Function : MATLAB Function  TreatAsAtomicUnit=on
      settings: PermitHierarchicalResolution=ParametersOnly
  MATLAB Function1 : MATLAB Function  TreatAsAtomicUnit=on
      settings: PermitHierarchicalResolution=ParametersOnly
  MATLAB Function2 : MATLAB Function  TreatAsAtomicUnit=on
      settings: PermitHierarchicalResolution=ParametersOnly
  MATLAB Function3 : MATLAB Function  Commented=on  TreatAsAtomicUnit=on
      settings: PermitHierarchicalResolution=ParametersOnly
  MATLAB Function4 : MATLAB Function  TreatAsAtomicUnit=on
      settings: PermitHierarchicalResolution=ParametersOnly
  Saturation : Saturate  UpperLimit=[1.03 2.5 0.98]'  LowerLimit=-[1.03 2.5 0.98]'
  Scope : Scope
      settings: TimeRange=auto  ShowLegends=on  MaxDataPoints=5000  SaveToWorkspace=off  YMin=-3.125  YMax=3.125  SampleTime=-1
  Scope1 : Scope
      settings: TimeRange=auto  MaxDataPoints=5000  SaveToWorkspace=off  SaveName=ScopeData2  YMin=-4361622909727543.00000  YMax=330140861095278.5  SampleTime=-1
  Scope2 : Scope
      settings: TimeRange=auto  MaxDataPoints=5000  SaveToWorkspace=off  SaveName=ScopeData3  YMin=-65.86026  YMax=75.79879  SampleTime=-1
  kinetics : MATLAB Function  TreatAsAtomicUnit=on
      settings: PermitHierarchicalResolution=ParametersOnly
  new_nu : Outport
  wires:
  eta_d_s/1 -> MATLAB Function1/3(eta_d_s), MATLAB Function4/4(eta_d_s)
  U_s/1 -> MATLAB Function4/6(U_s)
  eta_d/1 -> MATLAB Function2/1(eta_d), MATLAB Function1/2(eta_d)
  eta/1 -> MATLAB Function1/1(eta), MATLAB Function2/2(eta), MATLAB Function4/3(eta)
  MATLAB Function/1(tau) -> Scope2/1, Saturation/1
  K_p1/1 -> MATLAB Function3/1(K_p)
  MATLAB Function4/1(alpha_1_dot) -> MATLAB Function/2(alpha_dot)
  MATLAB Function1/1(z_1_dot) -> MATLAB Function4/2(z_1_dot)
  K_p/1 -> MATLAB Function4/1(K_p)
  U_s_s/1 -> MATLAB Function4/7(U_s_s)
  eta_d_ss/1 -> MATLAB Function4/8(eta_d_ss)
  s_dot/1 -> MATLAB Function1/5(s_dot), MATLAB Function4/9(s_dot)
  MATLAB Function2/1(z_1) -> MATLAB Function/3(z_1)
  Integrator/1 -> new_nu/1
  kinetics/1(nu_dot) -> Integrator/1
  nu/1 -> Scope1/1, kinetics/2(nu), MATLAB Function/1(nu), MATLAB Function1/4(nu), MATLAB Function4/5(nu)
  Saturation/1 -> Scope/1, kinetics/1(tau)

== system CaseD_2/Line System 2-6/Kinematic model1 ==
  nu : Inport
  Integrator : Integrator  InitialCondition=initial_eta
  Product : Product  Multiplication=Matrix(*)
  Rotation matrix : MATLAB Function  TreatAsAtomicUnit=on
      settings: PermitHierarchicalResolution=ParametersOnly
  Selector : Selector  InputPortWidth=3  IndexOptions=Starting index (dialog)  Indices=3  OutputSizes=1
  "eta " : Outport
  wires:
  Product/1 -> Integrator/1  "eta_dot"
  Integrator/1 -> Selector/1, "eta "/1  "eta"
  nu/1 -> Product/2
  Rotation matrix/1(R) -> Product/1
  Selector/1 -> Rotation matrix/1(psi)

== system CaseD_2/Line System 2-6/Line Mapper ==
  "s " : Inport
  MATLAB Function : MATLAB Function  TreatAsAtomicUnit=on
      settings: PermitHierarchicalResolution=ParametersOnly
  Memory : Memory
  P_d : Constant  Value=P_d
  eta_d : Outport  PortDimensions=3
  eta_d_s : Outport  Port=2  PortDimensions=3
  wires:
  MATLAB Function/1(eta_d) -> eta_d/1
  MATLAB Function/2(eta_d_s) -> eta_d_s/1
  "s "/1 -> MATLAB Function/1(s)
  P_d/1 -> MATLAB Function/2(P_d)
  Memory/1 -> MATLAB Function/3(s_proc_old)
  MATLAB Function/3(s_proc) -> Memory/1

== system CaseD_2/Line System 2-6/Line Speed Gauge ==
  U_ref : Inport
  Constant : Constant  Value=P_d
  Line : MATLAB Function  TreatAsAtomicUnit=on
      settings: PermitHierarchicalResolution=ParametersOnly
  U_s : Outport
  wires:
  U_ref/1 -> Line/1(U_ref)
  Line/1(U_s) -> U_s/1
  Constant/1 -> Line/2(P_d)

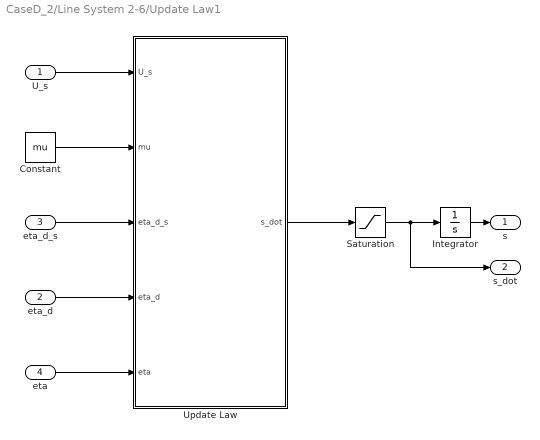
== system CaseD_2/Line System 2-6/Update Law1 ==
  U_s : Inport
  eta_d : Inport  Port=2
  eta_d_s : Inport  Port=3
  eta : Inport  Port=4
  Constant : Constant  Value=mu
  Integrator : Integrator  LimitOutput=on  UpperSaturationLimit=1  LowerSaturationLimit=0
  Saturation : Saturate  UpperLimit=inf  LowerLimit=0
  Update Law : MATLAB Function  TreatAsAtomicUnit=on
      settings: PermitHierarchicalResolution=ParametersOnly
  s : Outport
  s_dot : Outport  Port=2
  wires:
  U_s/1 -> Update Law/1(U_s)
  Constant/1 -> Update Law/2(mu)
  eta_d_s/1 -> Update Law/3(eta_d_s)
  eta_d/1 -> Update Law/4(eta_d)
  Integrator/1 -> s/1
  eta/1 -> Update Law/5(eta)
  Update Law/1(s_dot) -> Saturation/1
  Saturation/1 -> s_dot/1, Integrator/1

== system CaseD_2/Line System 3/Control law ==
  eta : Inport
  U_s : Inport  Port=2
  eta_d_s : Inport  Port=3
  eta_d : Inport  Port=4
  Control Law : MATLAB Function  TreatAsAtomicUnit=on
      settings: PermitHierarchicalResolution=ParametersOnly
  K_p : Constant  Value=K_p
  Scope : Scope
      settings: TimeRange=auto  MaxDataPoints=5000  SaveToWorkspace=off  SaveName=ScopeData3  YMin=-10576.35102  YMax=10326.26692  SampleTime=-1
  nu : Outport
  wires:
  K_p/1 -> Control Law/1(K_p)
  Control Law/1(nu) -> nu/1
  eta_d_s/1 -> Control Law/4(eta_d_s)
  U_s/1 -> Control Law/5(U_s)
  eta_d/1 -> Control Law/3(eta_d)
  eta/1 -> Control Law/2(eta)
  Control Law/2(z_1) -> Scope/1

== system CaseD_2/Line System 3/Kinematic model ==
  nu : Inport
  Integrator : Integrator  InitialCondition=initial_eta_2
  Product : Product  Multiplication=Matrix(*)
  Rotation matrix : MATLAB Function  TreatAsAtomicUnit=on
      settings: PermitHierarchicalResolution=ParametersOnly
  Selector : Selector  InputPortWidth=3  IndexOptions=Starting index (dialog)  Indices=3  OutputSizes=1
  "eta " : Outport
  wires:
  Product/1 -> Integrator/1  "eta_dot"
  Integrator/1 -> Selector/1, "eta "/1  "eta"
  nu/1 -> Product/2
  Rotation matrix/1(R) -> Product/1
  Selector/1 -> Rotation matrix/1(psi)

== system CaseD_2/Line System 3/Line Mapper ==
  s : Inport
  MATLAB Function : MATLAB Function  TreatAsAtomicUnit=on
      settings: PermitHierarchicalResolution=ParametersOnly
  Memory : Memory
  P_d : Constant  Value=P_d
  eta_d : Outport  PortDimensions=3
  eta_d_s : Outport  Port=2  PortDimensions=3
  wires:
  MATLAB Function/1(eta_d) -> eta_d/1
  MATLAB Function/2(eta_d_s) -> eta_d_s/1
  s/1 -> MATLAB Function/1(s)
  P_d/1 -> MATLAB Function/3(P_d)
  Memory/1 -> MATLAB Function/2(s_proc_old)
  MATLAB Function/3(s_proc) -> Memory/1

== system CaseD_2/Line System 3/Line Speed Gauge ==
  U_ref : Inport
  Constant : Constant  Value=P_d
  Line : MATLAB Function  TreatAsAtomicUnit=on
      settings: PermitHierarchicalResolution=ParametersOnly
  U_s : Outport
  wires:
  U_ref/1 -> Line/1(U_ref)
  Line/1(U_s) -> U_s/1
  Constant/1 -> Line/2(P_d)

== system CaseD_2/Line System 3/Update Law ==
  U_s : Inport
  eta_d : Inport  Port=2
  eta_d_s : Inport  Port=3
  eta : Inport  Port=4
  Constant : Constant  Value=mu
  Integrator : Integrator  UpperSaturationLimit=1  LowerSaturationLimit=0
  Update Law : MATLAB Function  TreatAsAtomicUnit=on
      settings: PermitHierarchicalResolution=ParametersOnly
  s : Outport
  wires:
  U_s/1 -> Update Law/1(U_s)
  Constant/1 -> Update Law/2(mu)
  eta_d_s/1 -> Update Law/3(eta_d_s)
  eta_d/1 -> Update Law/4(eta_d)
  Update Law/1(s_dot) -> Integrator/1
  Integrator/1 -> s/1
  eta/1 -> Update Law/5(eta)

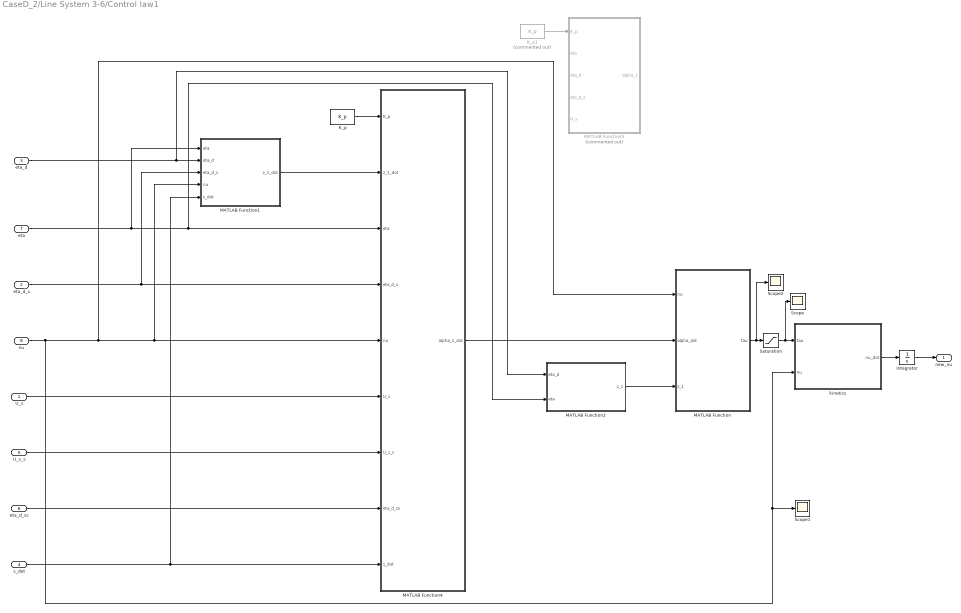
== system CaseD_2/Line System 3-6/Control law1 ==
  U_s : Inport
  eta_d_s : Inport  Port=2
  eta_d : Inport  Port=3
  s_dot : Inport  Port=4
  U_s_s : Inport  Port=5
  eta_d_ss : Inport  Port=6
  eta : Inport  Port=7
  nu : Inport  Port=8
  Integrator : Integrator  InitialCondition=[0 0 0]'
  K_p : Constant  Value=K_p
  K_p1 : Constant  Commented=on  Value=K_p
  MATLAB Function : MATLAB Function  TreatAsAtomicUnit=on
      settings: PermitHierarchicalResolution=ParametersOnly
  MATLAB Function1 : MATLAB Function  TreatAsAtomicUnit=on
      settings: PermitHierarchicalResolution=ParametersOnly
  MATLAB Function2 : MATLAB Function  TreatAsAtomicUnit=on
      settings: PermitHierarchicalResolution=ParametersOnly
  MATLAB Function3 : MATLAB Function  Commented=on  TreatAsAtomicUnit=on
      settings: PermitHierarchicalResolution=ParametersOnly
  MATLAB Function4 : MATLAB Function  TreatAsAtomicUnit=on
      settings: PermitHierarchicalResolution=ParametersOnly
  Saturation : Saturate  UpperLimit=[1.03 2.5 0.98]'  LowerLimit=-[1.03 2.5 0.98]'
  Scope : Scope
      settings: TimeRange=auto  ShowLegends=on  MaxDataPoints=5000  SaveToWorkspace=off  YMin=-3.125  YMax=3.125  SampleTime=-1
  Scope1 : Scope
      settings: TimeRange=auto  MaxDataPoints=5000  SaveToWorkspace=off  SaveName=ScopeData2  YMin=-4361622909727543.00000  YMax=330140861095278.5  SampleTime=-1
  Scope2 : Scope
      settings: TimeRange=auto  MaxDataPoints=5000  SaveToWorkspace=off  SaveName=ScopeData3  YMin=-65.86026  YMax=75.79879  SampleTime=-1
  kinetics : MATLAB Function  TreatAsAtomicUnit=on
      settings: PermitHierarchicalResolution=ParametersOnly
  new_nu : Outport
  wires:
  eta_d_s/1 -> MATLAB Function1/3(eta_d_s), MATLAB Function4/4(eta_d_s)
  U_s/1 -> MATLAB Function4/6(U_s)
  eta_d/1 -> MATLAB Function2/1(eta_d), MATLAB Function1/2(eta_d)
  eta/1 -> MATLAB Function1/1(eta), MATLAB Function2/2(eta), MATLAB Function4/3(eta)
  MATLAB Function/1(tau) -> Scope2/1, Saturation/1
  K_p1/1 -> MATLAB Function3/1(K_p)
  MATLAB Function4/1(alpha_1_dot) -> MATLAB Function/2(alpha_dot)
  K_p/1 -> MATLAB Function4/1(K_p)
  U_s_s/1 -> MATLAB Function4/7(U_s_s)
  eta_d_ss/1 -> MATLAB Function4/8(eta_d_ss)
  s_dot/1 -> MATLAB Function1/5(s_dot), MATLAB Function4/9(s_dot)
  MATLAB Function2/1(z_1) -> MATLAB Function/3(z_1)
  Integrator/1 -> new_nu/1
  kinetics/1(nu_dot) -> Integrator/1
  nu/1 -> Scope1/1, kinetics/2(nu), MATLAB Function/1(nu), MATLAB Function1/4(nu), MATLAB Function4/5(nu)
  Saturation/1 -> Scope/1, kinetics/1(tau)
  MATLAB Function1/1(z_1_dot) -> MATLAB Function4/2(z_1_dot)

== system CaseD_2/Line System 3-6/Kinematic model ==
  nu : Inport
  Integrator : Integrator  InitialCondition=initial_eta_2
  Product : Product  Multiplication=Matrix(*)
  Rotation matrix : MATLAB Function  TreatAsAtomicUnit=on
      settings: PermitHierarchicalResolution=ParametersOnly
  Selector : Selector  InputPortWidth=3  IndexOptions=Starting index (dialog)  Indices=3  OutputSizes=1
  "eta " : Outport
  wires:
  Product/1 -> Integrator/1  "eta_dot"
  Integrator/1 -> Selector/1, "eta "/1  "eta"
  nu/1 -> Product/2
  Rotation matrix/1(R) -> Product/1
  Selector/1 -> Rotation matrix/1(psi)

== system CaseD_2/Line System 3-6/Line Mapper ==
  s : Inport
  MATLAB Function : MATLAB Function  TreatAsAtomicUnit=on
      settings: PermitHierarchicalResolution=ParametersOnly
  Memory : Memory
  P_d : Constant  Value=P_d
  eta_d : Outport  PortDimensions=3
  eta_d_s : Outport  Port=2  PortDimensions=3
  wires:
  MATLAB Function/1(eta_d) -> eta_d/1
  MATLAB Function/2(eta_d_s) -> eta_d_s/1
  s/1 -> MATLAB Function/1(s)
  P_d/1 -> MATLAB Function/3(P_d)
  Memory/1 -> MATLAB Function/2(s_proc_old)
  MATLAB Function/3(s_proc) -> Memory/1

== system CaseD_2/Line System 3-6/Line Speed Gauge ==
  U_ref : Inport
  Constant : Constant  Value=P_d
  Line : MATLAB Function  TreatAsAtomicUnit=on
      settings: PermitHierarchicalResolution=ParametersOnly
  U_s : Outport
  wires:
  U_ref/1 -> Line/1(U_ref)
  Line/1(U_s) -> U_s/1
  Constant/1 -> Line/2(P_d)

== system CaseD_2/Line System 3-6/Update Law ==
  U_s : Inport
  eta_d : Inport  Port=2
  eta_d_s : Inport  Port=3
  eta : Inport  Port=4
  Constant : Constant  Value=mu
  Integrator : Integrator  UpperSaturationLimit=1  LowerSaturationLimit=0
  Update Law : MATLAB Function  TreatAsAtomicUnit=on
      settings: PermitHierarchicalResolution=ParametersOnly
  s : Outport
  s_dot : Outport  Port=2
  wires:
  U_s/1 -> Update Law/1(U_s)
  Constant/1 -> Update Law/2(mu)
  eta_d_s/1 -> Update Law/3(eta_d_s)
  eta_d/1 -> Update Law/4(eta_d)
  Update Law/1(s_dot) -> s_dot/1, Integrator/1
  Integrator/1 -> s/1
  eta/1 -> Update Law/5(eta)

== matlab function CaseD_2/Line System 3/Line Mapper/MATLAB Function ==
  data: s input; s_proc_old input; eta_d output; eta_d_s output; P_d input; s_proc output
function [eta_d, eta_d_s, s_proc] = linify(s, s_proc_old, P_d)
s = 1 - abs(mod(s, 2) - 1);
p_d = s.*[P_d(2, 1) - P_d(1, 1); P_d(2, 2) - P_d(1, 2)] + [P_d(1, 1); P_d(1, 2)];
psi_d = atan2(P_d(2, 2) - P_d(1, 2), P_d(2, 1) - P_d(1, 1));
if s_proc_old - s < 0
    psi_d = pi - psi_d;
end
p_d_s = [P_d(2, 1) - P_d(1, 1); P_d(2, 2) - P_d(1, 2)];
psi_d_s = 0;

eta_d = zeros(3, 1);
eta_d_s = zeros(3, 1);
eta_d = [p_d; psi_d];
eta_d_s = [p_d_s; psi_d_s];

s_proc = s;

== matlab function CaseD_2/Ellipse System/Kinematic model/MATLAB Function ==
  data: eta input; eta output
function eta = normalize(eta)
eta(3) = angdiff(0, eta(3));

== matlab function CaseD_2/Line System 3/Control law/Control Law ==
  data: K_p input; nu output; eta input; eta_d input; eta_d_s input; U_s input; z_1 output
function [nu, z_1] = control_law(K_p, eta, eta_d, eta_d_s, U_s)
psi = eta(3);
R = [cos(psi) -sin(psi) 0;
     sin(psi) cos(psi)  0;
     0        0         1];
 
 z_1_a = eta - eta_d;
% Here is where our eta_d would jump because of the parametrization.
% Instead of doing something hacky, we can redefine the control
% law such that it has the exact same gain.
% To compute the angular difference, we use angdiff:
z_1_psi = angdiff(eta_d(3), eta(3));
z_1_a(3) = z_1_psi;
z_1 = R'*z_1_a;
nu = -K_p*z_1 + R'*eta_d_s*U_s;

== matlab function CaseD_2/Line System 2/Control law/Control Law ==
  data: K_p input; nu output; eta input; eta_d input; eta_d_s input; U_s input; z_1 output
function [nu, z_1] = control_law(K_p, eta, eta_d, eta_d_s, U_s)
psi = eta(3);
R = [cos(psi) -sin(psi) 0;
     sin(psi) cos(psi)  0;
     0        0         1];
 
 z_1_a = eta - eta_d;
% Here is where our eta_d would jump because of the parametrization.
% Instead of doing something hacky, we can redefine the control
% law such that it has the exact same gain.
% To compute the angular difference, we use angdiff:
z_1_psi = angdiff(eta_d(3), eta(3));
z_1_a(3) = z_1_psi;
z_1 = R'*z_1_a;
nu = -K_p*z_1 + R'*eta_d_s*U_s;

== matlab function CaseD_2/Line System 1/Update Law/Update Law ==
  data: U_s input; s_dot output; mu input; eta_d_s input; eta_d input; eta input
function s_dot = update(U_s, mu, eta_d_s, eta_d, eta)
diff = eta - eta_d;
diff(3) = angdiff(eta_d(3), eta(3)); % Order is important here
s_dot = U_s - mu/norm(eta_d_s) * -diff' * eta_d_s;

== matlab function CaseD_2/Line System 1/Line Speed Gauge/Line ==
  data: U_ref input; U_s output; P_d input
function U_s = line(U_ref, P_d)
U_s = U_ref / sqrt(sum((P_d(:,2)-P_d(:,1)).^2));

== matlab function CaseD_2/Ellipse System/Control law/Control Law ==
  data: K_p input; nu output; eta input; eta_d input; eta_d_s input; U_s input; z_1 output
function [nu, z_1] = control_law(K_p, eta, eta_d, eta_d_s, U_s)
psi = eta(3);
R = [cos(psi) -sin(psi) 0;
     sin(psi) cos(psi)  0;
     0        0         1];
 
 z_1_a = eta - eta_d;
% Here is where our eta_d would jump because of the parametrization.
% Instead of doing something hacky, we can redefine the control
% law such that it has the exact same gain.
% To compute the angular difference, we use angdiff:
z_1_psi = angdiff(eta_d(3), eta(3));
z_1_a(3) = z_1_psi;
z_1 = R'*z_1_a;
nu = -K_p*z_1 + R'*eta_d_s*U_s;

== matlab function CaseD_2/Line System 1/Kinematic model/Rotation matrix ==
  data: psi input; R output
function R = rotation(psi)
R = [cos(psi) -sin(psi) 0;
     sin(psi) cos(psi)  0;
     0        0         1];

== matlab function CaseD_2/Ellipse System/Kinematic model/Rotation matrix ==
  data: psi input; R output
function R = rotation(psi)
R = [cos(psi) -sin(psi) 0;
     sin(psi) cos(psi)  0;
     0        0         1];

== matlab function CaseD_2/Line System 1/Control law/Control Law ==
  data: K_p input; nu output; eta input; eta_d input; eta_d_s input; U_s input; z_1 output
function [nu, z_1] = control_law(K_p, eta, eta_d, eta_d_s, U_s)
psi = eta(3);
R = [cos(psi) -sin(psi) 0;
     sin(psi) cos(psi)  0;
     0        0         1];
 
 z_1_a = eta - eta_d;
% Here is where our eta_d would jump because of the parametrization.
% Instead of doing something hacky, we can redefine the control
% law such that it has the exact same gain.
% To compute the angular difference, we use angdiff:
z_1_psi = angdiff(eta_d(3), eta(3));
z_1_a(3) = z_1_psi;
z_1 = R'*z_1_a;
nu = -K_p*z_1 + R'*eta_d_s*U_s;
% a = nu - tau
% We will have to compute tau here when using the system together with the
% kinematics

== matlab function CaseD_2/Ellipse System/Ellipse Speed Gauge/Ellipse ==
  data: U_ref input; s input; U_s output; r input
function U_s = ellipse(U_ref, s, r)
U_s = U_ref / sqrt((r(1)*sin(s))^2 + (r(2)*cos(s))^2);

== matlab function CaseD_2/Ellipse System/Update Law/Update Law ==
  data: U_s input; s_dot output; mu input; eta_d_s input; eta_d input; eta input
function s_dot = update(U_s, mu, eta_d_s, eta_d, eta)
diff = eta - eta_d;
diff(3) = angdiff(eta_d(3), eta(3)); % Order is important here
s_dot = U_s - mu/norm(eta_d_s) * -diff' * eta_d_s;

== matlab function CaseD_2/MATLAB Function1 ==
  data: eta input; z_1_dot output; eta_d input; eta_d_s input; nu input; s_dot input
function z_1_dot = derive_z_1(eta, eta_d, eta_d_s, nu, s_dot)
r = nu(3);
S = [0 -r 0; r 0 0; 0 0 0];

psi = eta(3);
R = [cos(psi) -sin(psi) 0;
     sin(psi) cos(psi)  0;
     0        0         1];
 
 z_1_a = eta - eta_d;
% Here is where our eta_d would jump because of the parametrization.
% Instead of doing something hacky, we can redefine the control
% law such that it has the exact same gain.
% To compute the angular difference, we use angdiff:
z_1_psi = angdiff(eta_d(3), eta(3));
z_1_a(3) = z_1_psi;
z_1 = R'*z_1_a;
z_1_dot = S'*z_1 + nu - R'*eta_d_s*s_dot;

== matlab function CaseD_2/Line System 1/Line Mapper/MATLAB Function ==
  data: s input; eta_d output; eta_d_s output; P_d input
function [eta_d, eta_d_s] = linify(s, P_d)
p_d = [P_d(2,1) - P_d(1,1); P_d(2,2) - P_d(1,2)]*s + [P_d(1,1); P_d(1,2)];
psi_d = atan2(P_d(2,2) - P_d(1,2), P_d(2,1) - P_d(1,1));

p_d_s = [P_d(2,1) - P_d(1,1); P_d(2,2) - P_d(1,2)];
psi_d_s = 0;

eta_d = [p_d; psi_d];
eta_d_s = [p_d_s; psi_d_s];

== matlab function CaseD_2/Ellipse System 4-6/Ellipse Mapper /Ellipse Mapper ==
  data: s input; eta_d output; C input; R input; eta_d_s output; eta_d_ss output
function [eta_d, eta_d_s, eta_d_ss] = ellipse(s, C, R)
rx = R(1,1);
ry = R(2,2);

eta_d = [rx*cos(s)+C(1);
         ry*sin(s)+C(2);
         %0;];
         atan2(ry*cos(s), -rx*sin(s))]; % + floor((s+2*pi-pi/2)/2/pi)*2*pi];

eta_d_s = [-rx*sin(s);
           ry*cos(s);
           %0;];
           rx*ry/(ry^2*cos(s)^2+rx^2*sin(s)^2)];
eta_d_ss = [-rx*cos(s);
            -ry*sin(s);
            -2*(rx^2*cos(s)*sin(s) - ry^2*cos(s)*sin(s))*rx*ry/(ry^2*cos(s)^2 + rx^2*sin(s)^2)^2];

== matlab function CaseD_2/Line System 2/Kinematic model/Rotation matrix ==
  data: psi input; R output
function R = rotation(psi)
R = [cos(psi) -sin(psi) 0;
     sin(psi) cos(psi)  0;
     0        0         1];

== matlab function CaseD_2/Line System 2/Line Mapper/MATLAB Function ==
  data: s input; P_d input; s_proc_old input; eta_d output; eta_d_s output; s_proc output
function [eta_d, eta_d_s, s_proc] = linify(s, P_d, s_proc_old)
s = 1 - abs(mod(s, 2) - 1);
p_d = s.*[P_d(2, 1) - P_d(1, 1); P_d(2, 2) - P_d(1, 2)] + [P_d(1, 1); P_d(1, 2)];
psi_d = atan2(P_d(2, 2) - P_d(1, 2), P_d(2, 1) - P_d(1, 1));
if s_proc_old - s < 0
    psi_d = pi - psi_d;
end
p_d_s = [P_d(2, 1) - P_d(1, 1); P_d(2, 2) - P_d(1, 2)];
psi_d_s = 0;

eta_d = zeros(3, 1);
eta_d_s = zeros(3, 1);
eta_d = [p_d; psi_d];
eta_d_s = [p_d_s; psi_d_s];

s_proc = s;

== matlab function CaseD_2/Line System 2/Line Speed Gauge/Line ==
  data: U_ref input; U_s output; P_d input
function U_s = line(U_ref, P_d)
U_s = U_ref / sqrt(sum((P_d(:,2)-P_d(:,1)).^2));
